simulink model "index_stm32g4"  (R2024b)
settings: Solver=FixedStepAuto  StartTime=0.0  StopTime=10.0  RelTol=1e-3  EnableMultiTasking=on
libraries: stm32f4xxblockslib x5, filckering_filter x5, stm32g4xxblockslib x2, stm32blockslib x2, root x1, usart_to_cmd x1, state_to_relay x1
settings Model: STM32="{\"UARTRead\":{\"ID\":\"index_stm32g4:12\"},\"UARTWrite\":{\"ID\":\"index_stm32g4:13\"},\"DigitalPortRead\":[{\"ID\":\"index_stm32g4:20\"},{\"ID\":\"index_stm32g4:22\"},{\"ID\":\"index_stm32g4:23\"}],\"DigitalPortWrite\":[{\"ID\":\"index_stm32g4:21\"},{\"ID\":\"index_stm32g4:27\"}],\"PWMOutput\":[{\"ID\":\"index_stm32g4:25\"},{\"ID\":\"index_stm32g4:26\"}]}"  Creator=mainuser  LastModifiedBy=mainuser
settings OptimizationCC: DefaultParameterBehavior=Inlined  EnhancedBackFolding=on  PassReuseOutputArgsAs=Individual arguments  ZeroExternalMemoryAtStartup=off  ZeroInternalMemoryAtStartup=off  MaxStackSize=512  OptimizeBlockOrder=speed  DifferentSizesBufferReuse=on  OptimizationCustomize=off  EfficientTunableParamExpr=on
settings DebuggingCC: ParameterTunabilityLossMsg=error
settings HardwareCC: ProdBitPerPointer=32  ProdBitPerSizeT=32  ProdBitPerPtrDiffT=32  ProdLargestAtomicInteger=Long  ProdLargestAtomicFloat=Double  ProdWordSize=32  ProdLongLongMode=on  ProdHWDeviceType=ARM Compatible->ARM Cortex-M
settings SFSimCC: MATLABDynamicMemAlloc=off
settings RTWCC: Description=Embedded Coder  SystemTargetFile=ert.tlc  HardwareBoard=STM32G4xx Based  TemplateMakefile=ert_default_tmf  Toolchain=GNU Tools for ARM Embedded Processors
settings CodeAppCC: ForceParamTrailComments=on  IgnoreCustomStorageClasses=off  OperatorAnnotations=on  SimulinkDataObjDesc=on  SFDataObjDesc=on  InsertBlockDesc=on
settings ERTTargetCC: TargetLangStandard=C99 (ISO)  CodeReplacementLibrary=ARM Cortex-M  SupportVariableSizeSignals=on  ExtModeTransport=3  ExtModeStaticAlloc=on  ExtModeStaticAllocSize=2048  ExtModeMexFile=ext_xcp  ExtModeIntrfLevel=Level2 - Open

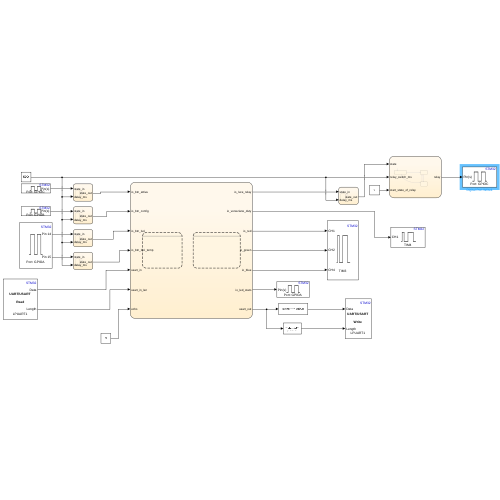
[thumbnail: Simulink's stored preview of the top-level diagram]
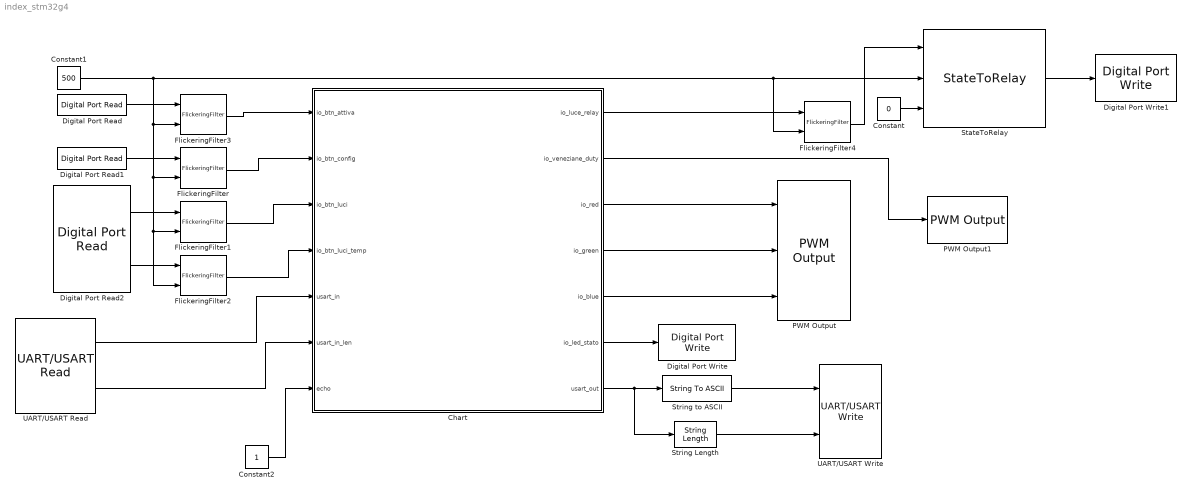
== system index_stm32g4 ==
  Chart : Stateflow chart  TreatAsAtomicUnit=on
      settings: PortSchema="{\"entries\":[{\"content\":{\"sides\":[{\"content\":{\"connectorIds\":[\"In1\",\"In2\",\"In3\",\"In4\",\"In6\",\"In7\",\"In5\"]},\"type\":\"ConnectorPlacement.EquallySpacedRectSide\",\"uuid\":\"0880ae90-b5dc-4c25-abd1-4f82521f475c\"},{\"content\":{\"connectorIds\":[\"Out1\",\"Out2\",\"Out3\",\"Out4\",\"Out5\",\"Out6\",\"Out7\"],\"side\":\"RIGHT\"},\"type\":\"ConnectorPlacement.EquallySpacedRectSide\",\"uuid\":\"1bbd8fe6-dda4-4d1c-809c-50b56dc39330\"},{\"content\":{\"side\":\"TOP\"},\"type\":\"ConnectorPlacement.EquallySpacedRectSide\",\"uuid\":\"5bacfcdb-1fe0-4905-b5b0-9d63287c1023\"}]},\"type\":\"ConnectorPlacement.EquallySpacedConnector\",\"uuid\":\"a9989c3c-7f31-4978-988a-0bacdc663247\"}],\"packageUris\":[\"http://schema.mathworks.com/mf0/Connector/R2020b\"],\"version\":\"1.0\"}"
  Constant : Constant  Value=0  OutDataTypeStr=boolean
  Constant1 : Constant  Value=500  OutDataTypeStr=uint32
  Constant2 : Constant  OutDataTypeStr=boolean
  Digital Port Read : stm32f4xxblockslib/Digital Port Read  PortName=GPIOC  PinNumber=[13]  ReadOperation=on  IOAsArray=on  SampleTime=-1  EnableSimPort=off  hoistedMaskSrc=ECSoC/ECSimCodegen/Digital Port Read
      settings: LibrarySourceBlock=stm32g4xxblockslib/Digital Port Read
  Digital Port Read1 : stm32f4xxblockslib/Digital Port Read  PortName=GPIOB  PinNumber=[0]  ReadOperation=on  IOAsArray=on  SampleTime=-1  EnableSimPort=off  hoistedMaskSrc=ECSoC/ECSimCodegen/Digital Port Read
      settings: LibrarySourceBlock=stm32g4xxblockslib/Digital Port Read
  Digital Port Read2 : stm32f4xxblockslib/Digital Port Read  PortName=GPIOA  PinNumber=[14,15]  ReadOperation=on  IOAsArray=off  SampleTime=-1  EnableSimPort=off  hoistedMaskSrc=ECSoC/ECSimCodegen/Digital Port Read
      settings: LibrarySourceBlock=stm32g4xxblockslib/Digital Port Read
  Digital Port Write : stm32f4xxblockslib/Digital Port Write  PortName=GPIOA  PinNumber=[5]  ReadOperation=off  IOAsArray=on  EnableSimPort=off  hoistedMaskSrc=ECSoC/ECSimCodegen/Digital Port Write
      settings: LibrarySourceBlock=stm32g4xxblockslib/Digital Port Write
  Digital Port Write1 : stm32f4xxblockslib/Digital Port Write  PortName=GPIOC  PinNumber=[2]  ReadOperation=off  IOAsArray=on  EnableSimPort=off  hoistedMaskSrc=ECSoC/ECSimCodegen/Digital Port Write
      settings: LibrarySourceBlock=stm32g4xxblockslib/Digital Port Write
  FlickeringFilter{,1..4} (5 alike) : filckering_filter/FlickeringFilter  SystemSampleTime=-1  VariantActivationTime=update diagram  AllowFlexibleInterface=on  Latency=0  AutoFrameSizeCalculation=off
  PWM Output : stm32g4xxblockslib/PWM Output  TimerModule=TIM3  DutycycleUnits=Percentage  EnableChannel1=on  EnableChannel2=on  EnableChannel3=off  EnableChannel4=on  EnableChannel5=off  EnableChannel6=off  EnableCounterInput=off  EnableMainOutputInput=off  EnableFrequencyInput=off  SetRCAfterCE=off  OutputDirection=off  OutputMainOutputEnableStatus=off  SampleTime=0.1  EnableSimPort=off  EnableUpdateEvent=off  EnableCaptureCompare1Event=off  EnableCaptureCompare2Event=off  EnableCaptureCompare3Event=off  EnableCaptureCompare4Event=off  EnableTriggerEvent=off  EnableBreakEvent=off  EnableBreakEvent2=off  ProcessorFamily=STM32G4  hoistedMaskSrc=ECSoC/ECSimCodegen/PWM Output
  PWM Output1 : stm32g4xxblockslib/PWM Output  TimerModule=TIM4  DutycycleUnits=Percentage  EnableChannel1=on  EnableChannel2=off  EnableChannel3=off  EnableChannel4=off  EnableChannel5=off  EnableChannel6=off  EnableCounterInput=off  EnableMainOutputInput=off  EnableFrequencyInput=off  SetRCAfterCE=off  OutputDirection=off  OutputMainOutputEnableStatus=off  SampleTime=0.1  EnableSimPort=off  EnableUpdateEvent=off  EnableCaptureCompare1Event=off  EnableCaptureCompare2Event=off  EnableCaptureCompare3Event=off  EnableCaptureCompare4Event=off  EnableTriggerEvent=off  EnableBreakEvent=off  EnableBreakEvent2=off  ProcessorFamily=STM32G4  hoistedMaskSrc=ECSoC/ECSimCodegen/PWM Output
  StateToRelay : state_to_relay/StateToRelay  SystemSampleTime=-1  VariantActivationTime=update diagram  AllowFlexibleInterface=on  Latency=0  AutoFrameSizeCalculation=off
  String Length : StringLength
  String to ASCII : StringToASCII  OutputVectorSize=127
  UART/USART Read : stm32blockslib/UART//USART Read  UARTModule=LPUART1  DataType=uint8  DataLength=1  BlockingMode=off  BlockingTimeout=0.1  OutputLength=on  OutputStatus=off  SampleTime=-1
      settings: LibrarySourceBlock=stm32g4xxblockslib/UART//USART Read
  UART/USART Write : stm32blockslib/UART//USART Write  UARTModule=LPUART1  LengthOfDataToSend=on  BlockingMode=off  BlockingTimeout=0.1  OutputStatus=off
      settings: LibrarySourceBlock=stm32g4xxblockslib/UART//USART Write
  wires:
  FlickeringFilter/1 -> Chart/2(io_btn_config)
  FlickeringFilter1/1 -> Chart/3(io_btn_luci)
  FlickeringFilter2/1 -> Chart/4(io_btn_luci_temp)
  FlickeringFilter3/1 -> Chart/1(io_btn_attiva)
  Chart/1(io_luce_relay) -> FlickeringFilter4/1
  FlickeringFilter4/1 -> StateToRelay/1
  Constant/1 -> StateToRelay/3
  Constant1/1 -> FlickeringFilter4/2, StateToRelay/2, FlickeringFilter2/2, FlickeringFilter1/2, FlickeringFilter/2, FlickeringFilter3/2
  UART/USART Read/2 -> Chart/7(usart_in_len)
  UART/USART Read/1 -> Chart/6(usart_in)
  Chart/7(usart_out) -> String Length/1, String to ASCII/1
  String to ASCII/1 -> UART/USART Write/1
  String Length/1 -> UART/USART Write/2
  Constant2/1 -> Chart/5(echo)
  Digital Port Read/1 -> FlickeringFilter3/1
  Chart/6(io_led_stato) -> Digital Port Write/1
  Digital Port Read1/1 -> FlickeringFilter/1
  Digital Port Read2/1 -> FlickeringFilter1/1
  Digital Port Read2/2 -> FlickeringFilter2/1
  Chart/3(io_red) -> PWM Output/1
  Chart/4(io_green) -> PWM Output/2
  Chart/5(io_blue) -> PWM Output/3
  Chart/2(io_veneziane_duty) -> PWM Output1/1
  StateToRelay/1 -> Digital Port Write1/1

== stateflow chart index_stm32g4/Chart ==
  state UsartToCMD [parallel]
    settings: executionOrder=1
  state Root [parallel]
    settings: executionOrder=2
  data: toconf_val function_output; output_val function_input; toconf_invio function_output; output_invio function_input; io_cmd_out function_output; io_cmd_in_invio function_input; io_cmd_in_valore function_input; io_cmd_out_invio function_output; io_luce_relay output boolean size=1; io_veneziane_duty output double size=1; io_btn_attiva input boolean size=1; io_btn_config input boolean size=1; io_btn_luci input boolean size=1; io_btn_luci_temp input boolean size=1; echo input boolean size=1; io_red output double size=1; io_green output double size=1; io_blue output double size=1; io_led_stato output boolean size=1; toconf_invio local boolean size=1; toconf_valore local uint8; io_cmd_out local string; usart_in input uint8 size=1; usart_in_len input uint32 size=1; usart_out output string; output_invio local boolean size=1
